simulink model "kinova"  (R2021a)
settings: Solver=FixedStepDiscrete  StartTime=0.0  StopTime=Inf  RelTol=1e-3
undefined symbols (not defined in the file): duration, gripper_finger1_joint, gripper_finger2_joint, index, joint_1, joint_2, joint_4, joint_name, model_name, my_gen3, position, velocity
libraries: robotgazebolib x28, simulink x5, rllib x1, robotlib x1
settings Model: Creator=tareksaid  LastModifiedBy=uthm

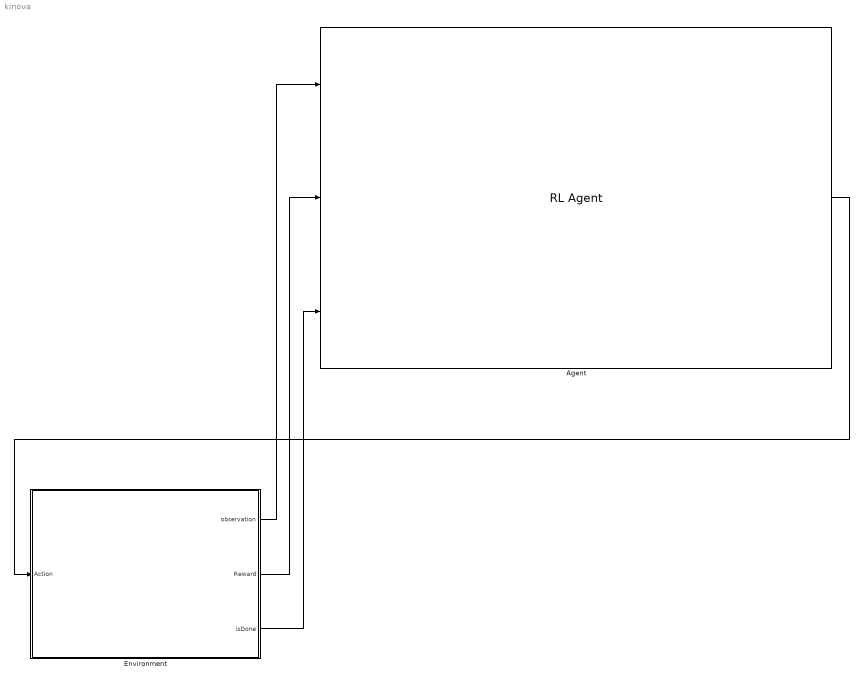
== system kinova ==
  Agent : rllib/RL Agent  Agent=Agent  ExternalActionAsInput=off  ProvideCumRwd=off  TreatAsDirectFeedthrough=on
  Environment : Subsystem
  wires:
  Environment/2(Reward) -> Agent/2
  Environment/1(observation) -> Agent/1
  Environment/3(isDone) -> Agent/3
  Agent/1 -> Environment/1(Action)

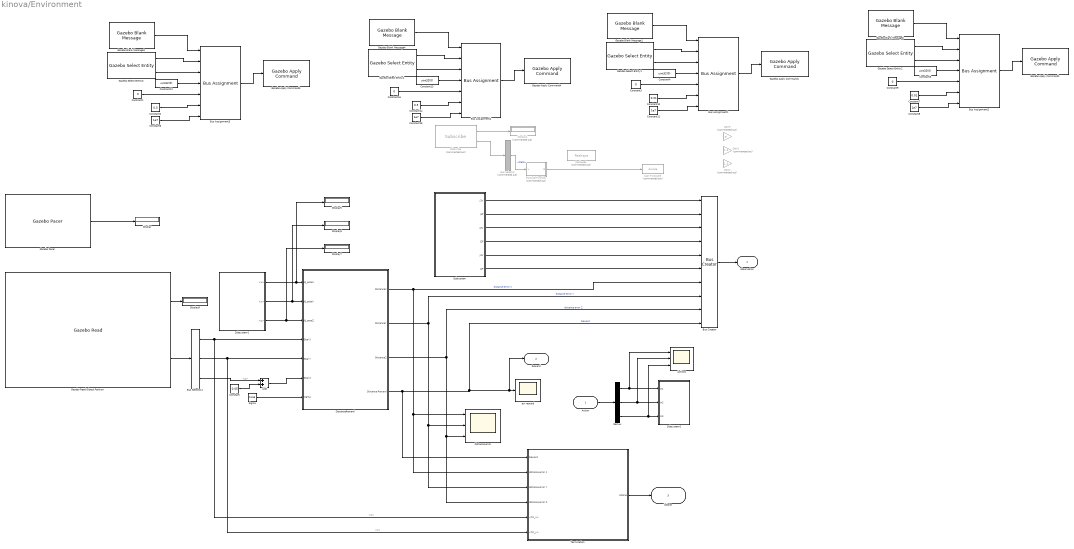
== system kinova/Environment ==
  Action : Inport
  Actions : Scope  NumInputPorts=3
  Add : Sum
  Bus Assignment1 : BusAssignment  AssignedSignals=model_name,joint_name,index,position,duration.seconds,duration.nano_seconds
  Bus Assignment2 : BusAssignment  AssignedSignals=model_name,joint_name,index,position,duration.seconds,duration.nano_seconds
  Bus Assignment3 : BusAssignment  AssignedSignals=model_name,joint_name,index,velocity,duration.seconds,duration.nano_seconds
  Bus Assignment4 : BusAssignment  AssignedSignals=model_name,joint_name,index,velocity,duration.seconds,duration.nano_seconds
  Bus Creator : BusCreator  Inputs=10
  Bus Selector : BusSelector  Commented=on  OutputSignals=Data
  Bus Selector4 : BusSelector  OutputSignals=position.x,position.y,position.z
  Cast To Double : DataTypeConversion  Commented=on  OutDataTypeStr=double
  Constant : Constant  Value=0.05
  Constant{1,3,9,16} (4 alike) : Constant  Value=0
  Constant10 : Constant  Value=0.01
  Constant{6,8,11,15} (4 alike) : Constant  Value=1e7
  Constant{4..5,12..13} (4 alike) : Constant  Value=uint32(0)
  Constant14 : Constant  Value=0.5
  Constant2 : Constant  Value=0.5
  Constant7 : Constant  Value=0.01
  Demux : Demux  Outputs=3
  Display{,5..8} (5 alike) : Display
  Display1 : Display  Commented=on
  Distance error : Scope  NumInputPorts=3
  DistanceReward : Subsystem
  Gain1 : Gain  Commented=on  Gain=1.3
  Gain2 : Gain  Commented=on  Gain=1.3
  Gain3 : Gain  Commented=on  Gain=pi
  Gazebo Apply Command1 : robotgazebolib/Gazebo Apply Command  cmdType=SetJointPosition  sampleTime=0.1
      settings: SourceProductBaseCode=RO
  Gazebo Apply Command2 : robotgazebolib/Gazebo Apply Command  cmdType=SetJointPosition  sampleTime=0.1
      settings: SourceProductBaseCode=RO
  Gazebo Apply Command3 : robotgazebolib/Gazebo Apply Command  cmdType=SetJointVelocity  sampleTime=0.1
      settings: SourceProductBaseCode=RO
  Gazebo Apply Command4 : robotgazebolib/Gazebo Apply Command  cmdType=SetJointVelocity  sampleTime=0.1
      settings: SourceProductBaseCode=RO
  Gazebo Blank Message1 : robotgazebolib/Gazebo Blank Message  msgType=SetJointPosition  sampleTime=0.1  busName='Gazebo_SL_Bus_gazebo_msgs_SetJointPosition'
      settings: SourceProductBaseCode=RO
  Gazebo Blank Message2 : robotgazebolib/Gazebo Blank Message  msgType=SetJointPosition  sampleTime=0.1  busName='Gazebo_SL_Bus_gazebo_msgs_SetJointPosition'
      settings: SourceProductBaseCode=RO
  Gazebo Blank Message3 : robotgazebolib/Gazebo Blank Message  msgType=SetJointVelocity  sampleTime=0.1  busName='Gazebo_SL_Bus_gazebo_msgs_SetJointVelocity'
      settings: SourceProductBaseCode=RO
  Gazebo Blank Message4 : robotgazebolib/Gazebo Blank Message  msgType=SetJointVelocity  sampleTime=0.1  busName='Gazebo_SL_Bus_gazebo_msgs_SetJointVelocity'
      settings: SourceProductBaseCode=RO
  Gazebo Pacer : robotgazebolib/Gazebo Pacer  ResetBehavior=Reset Gazebo simulation time and scene  SampleTime=0.1
      settings: SourceProductBaseCode=RO
  Gazebo Read Object Position : robotgazebolib/Gazebo Read  topicSource=From Gazebo  topic=/gazebo/ground_truth/world_pose/Yellow Can/link  messageType=gazebo_msgs/Pose  sampleTime=0.1
      settings: SourceProductBaseCode=RO
  Gazebo Select Entity1 : robotgazebolib/Gazebo Select Entity  modelElemName=my_gen3/gripper_finger1_joint  outputArraySize=128  OutputLabel=Joint  SelectType=Joint
      settings: SourceProductBaseCode=RO
  Gazebo Select Entity2 : robotgazebolib/Gazebo Select Entity  modelElemName=my_gen3/gripper_finger2_joint  outputArraySize=128  OutputLabel=Joint  SelectType=Joint
      settings: SourceProductBaseCode=RO
  Gazebo Select Entity3 : robotgazebolib/Gazebo Select Entity  modelElemName=my_gen3/gripper_finger1_joint  outputArraySize=128  OutputLabel=Joint  SelectType=Joint
      settings: SourceProductBaseCode=RO
  Gazebo Select Entity4 : robotgazebolib/Gazebo Select Entity  modelElemName=my_gen3/gripper_finger2_joint  outputArraySize=128  OutputLabel=Joint  SelectType=Joint
      settings: SourceProductBaseCode=RO
  MATLAB Function : MATLAB Function  Commented=on  TreatAsAtomicUnit=on
  Reshape1 : Reshape  Commented=on  OutputDimensionality=Customize  OutputDimensions=[10000,1]
  Sigma : Constant  Value=0.415
  Subscribe : robotlib/Subscribe  Commented=on  topicSource=Select from ROS network  topic=/camera/depth/image_raw  messageType=sensor_msgs/Image  SampleTime=-1  legacyBusStruct=off  messageQueueLength=1
  Subsystem : Subsystem
  Subsystem1 : Subsystem
  Subsystem2 : Subsystem
  Termination : Subsystem
  avr reward : Scope
  observation : Outport
  Reward : Outport  Port=2
  isDone : Outport  Port=3  VectorParamsAs1DForOutWhenUnconnected=off
  wires:
  Bus Creator/1 -> observation/1
  Termination/1(isDone) -> isDone/1
  Gazebo Pacer/1 -> Display/1
  DistanceReward/1(DistanceX) -> Bus Creator/7, Termination/2(distance error X), Distance error/1  "distance error X"
  Bus Selector4/2 -> Termination/6(<tin_y>), DistanceReward/5(Goal Y)  "<y>"
  DistanceReward/4(Distance Reward) -> Termination/1(Reward), Bus Creator/10, avr reward/1, Reward/1  "Reward"
  DistanceReward/2(DistanceY) -> Bus Creator/8, Termination/3(distance error Y), Distance error/2  "distance error Y"
  DistanceReward/3(DistanceZ) -> Bus Creator/9, Termination/4(distance error Z), Distance error/3  "distance error Z"
  Sigma/1 -> DistanceReward/7(sigma)
  Action/1 -> Demux/1
  Demux/2 -> Actions/2, Subsystem2/2(In2)
  Demux/3 -> Actions/3, Subsystem2/3(In3)
  Demux/1 -> Actions/1, Subsystem2/1(In1)
  Gazebo Read Object Position/1 -> Display8/1
  Gazebo Read Object Position/2 -> Bus Selector4/1
  Bus Selector4/1 -> Termination/5(<tin_x>), DistanceReward/4(Goal X)  "<x>"
  Subsystem/1(J1V) -> Bus Creator/1
  Subsystem/2(J1P) -> Bus Creator/2
  Subsystem/3(J2V) -> Bus Creator/3
  Subsystem/4(J2P) -> Bus Creator/4
  Subsystem/5(J4V) -> Bus Creator/5
  Subsystem/6(J4P) -> Bus Creator/6
  Subsystem1/2(<y>) -> Display6/1, DistanceReward/2(j8_poseY)
  Subsystem1/3(<z>) -> Display7/1, DistanceReward/3(j8_poseZ)
  Subsystem1/1(<x>) -> Display5/1, DistanceReward/1(j8_poseX)
  Subscribe/2 -> Bus Selector/1
  Bus Selector/1 -> MATLAB Function/1(u)  "<Data>"
  Subscribe/1 -> Display1/1
  MATLAB Function/1(D) -> Cast To Double/1
  Bus Selector4/3 -> Add/1  "<z>"
  Constant/1 -> Add/2
  Add/1 -> DistanceReward/6(Goal Z)
  Bus Assignment3/1 -> Gazebo Apply Command3/1
  Gazebo Select Entity3/2 -> Bus Assignment3/3
  Gazebo Select Entity3/1 -> Bus Assignment3/2
  Constant12/1 -> Bus Assignment3/4
  Constant16/1 -> Bus Assignment4/5
  Constant6/1 -> Bus Assignment3/7
  Constant2/1 -> Bus Assignment3/6
  Gazebo Blank Message3/1 -> Bus Assignment3/1
  Constant1/1 -> Bus Assignment3/5
  Bus Assignment4/1 -> Gazebo Apply Command4/1
  Constant15/1 -> Bus Assignment4/7
  Gazebo Blank Message4/1 -> Bus Assignment4/1
  Gazebo Select Entity4/1 -> Bus Assignment4/2
  Gazebo Select Entity4/2 -> Bus Assignment4/3
  Constant13/1 -> Bus Assignment4/4
  Constant14/1 -> Bus Assignment4/6
  Constant7/1 -> Bus Assignment2/6
  Constant5/1 -> Bus Assignment2/4
  Gazebo Select Entity2/2 -> Bus Assignment2/3
  Gazebo Select Entity2/1 -> Bus Assignment2/2
  Gazebo Blank Message2/1 -> Bus Assignment2/1
  Constant8/1 -> Bus Assignment2/7
  Bus Assignment2/1 -> Gazebo Apply Command2/1
  Constant3/1 -> Bus Assignment1/5
  Gazebo Blank Message1/1 -> Bus Assignment1/1
  Constant10/1 -> Bus Assignment1/6
  Constant11/1 -> Bus Assignment1/7
  Constant9/1 -> Bus Assignment2/5
  Constant4/1 -> Bus Assignment1/4
  Gazebo Select Entity1/1 -> Bus Assignment1/2
  Gazebo Select Entity1/2 -> Bus Assignment1/3
  Bus Assignment1/1 -> Gazebo Apply Command1/1

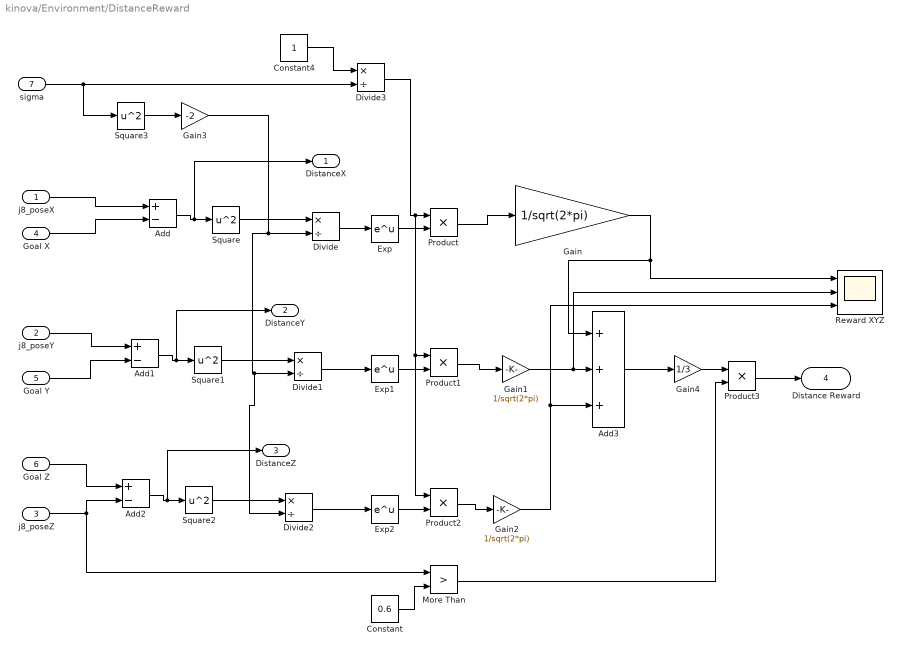
== system kinova/Environment/DistanceReward ==
  j8_poseX : Inport
  j8_poseY : Inport  Port=2
  j8_poseZ : Inport  Port=3
  Goal X : Inport  Port=4
  Goal Y : Inport  Port=5
  Goal Z : Inport  Port=6
  sigma : Inport  Port=7
  Add : Sum  Inputs=+-
  Add1 : Sum  Inputs=+-
  Add2 : Sum  Inputs=+-
  Add3 : Sum  Inputs=+++
  Constant : Constant  Value=0.6
  Constant4 : Constant
  Divide{,1..3} (4 alike) : Product  Inputs=*/
  Exp : Math  SaturateOnIntegerOverflow=on
  Exp1 : Math  SaturateOnIntegerOverflow=on
  Exp2 : Math  SaturateOnIntegerOverflow=on
  Gain : Gain  Gain=1/sqrt(2*pi)
  Gain1 : Gain  Gain=1/sqrt(2*pi)
  Gain2 : Gain  Gain=1/sqrt(2*pi)
  Gain3 : Gain  Gain=-2
  Gain4 : Gain  Gain=1/3
  More Than : RelationalOperator  Operator=>  OutDataTypeStr=boolean  RndMeth=Simplest
  Product{,1..3} (4 alike) : Product
  Reward XYZ : Scope  NumInputPorts=3
  Square{,1..3} (4 alike) : Math  Operator=square  SaturateOnIntegerOverflow=on
  DistanceX : Outport
  DistanceY : Outport  Port=2
  DistanceZ : Outport  Port=3
  Distance Reward : Outport  Port=4
  wires:
  Goal X/1 -> Add/2
  j8_poseX/1 -> Add/1
  Divide/1 -> Exp/1
  Square/1 -> Divide/1
  Add/1 -> DistanceX/1, Square/1
  Add1/1 -> Square1/1, DistanceY/1
  Square1/1 -> Divide1/1
  Divide1/1 -> Exp1/1
  j8_poseY/1 -> Add1/1
  Goal Y/1 -> Add1/2
  Divide2/1 -> Exp2/1
  Square2/1 -> Divide2/1
  Add2/1 -> DistanceZ/1, Square2/1
  Goal Z/1 -> Add2/1
  Gain1/1 -> Reward XYZ/2, Add3/2
  Gain/1 -> Add3/1, Reward XYZ/1
  Gain2/1 -> Add3/3, Reward XYZ/3
  Square3/1 -> Gain3/1
  Constant4/1 -> Divide3/1
  sigma/1 -> Divide3/2, Square3/1
  Exp/1 -> Product/2
  Exp1/1 -> Product1/2
  Exp2/1 -> Product2/2
  Divide3/1 -> Product2/1, Product1/1, Product/1
  Product/1 -> Gain/1
  Product1/1 -> Gain1/1
  Product2/1 -> Gain2/1
  Gain3/1 -> Divide/2, Divide2/2, Divide1/2
  Add3/1 -> Gain4/1
  More Than/1 -> Product3/2
  Constant/1 -> More Than/2
  j8_poseZ/1 -> More Than/1, Add2/2
  Gain4/1 -> Product3/1
  Product3/1 -> Distance Reward/1

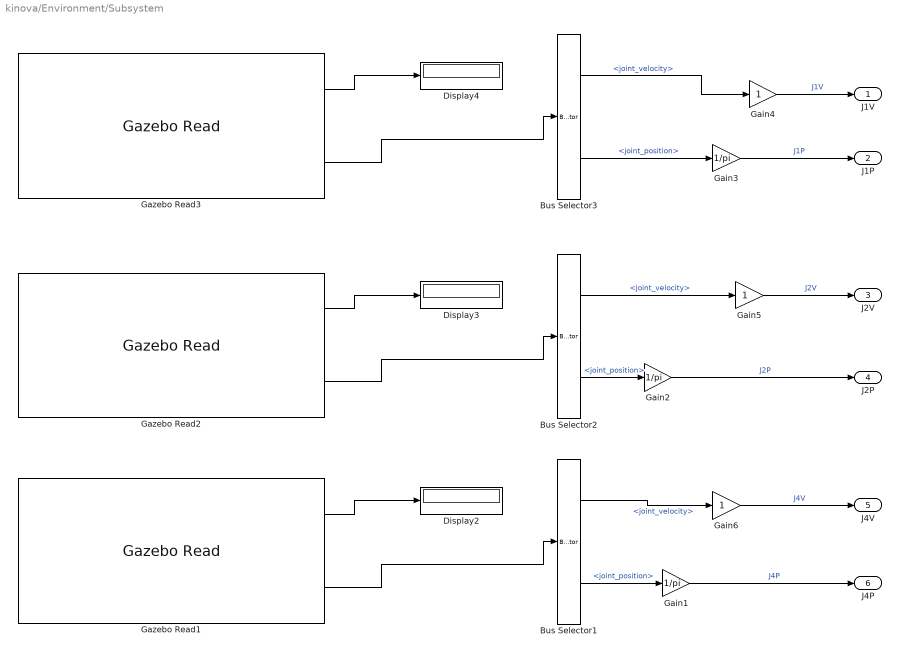
== system kinova/Environment/Subsystem ==
  Bus Selector1 : BusSelector  OutputSignals=joint_velocity,joint_position
  Bus Selector2 : BusSelector  OutputSignals=joint_velocity,joint_position
  Bus Selector3 : BusSelector  OutputSignals=joint_velocity,joint_position
  Display2 : Display
  Display3 : Display
  Display4 : Display
  Gain1 : Gain  Gain=1/pi
  Gain2 : Gain  Gain=1/pi
  Gain3 : Gain  Gain=1/pi
  Gain4 : Gain
  Gain5 : Gain
  Gain6 : Gain
  Gazebo Read1 : robotgazebolib/Gazebo Read  topicSource=From Gazebo  topic=/gazebo/ground_truth/joint_state/my_gen3/joint_4  messageType=gazebo_msgs/JointState  sampleTime=0.1
      settings: SourceProductBaseCode=RO
  Gazebo Read2 : robotgazebolib/Gazebo Read  topicSource=From Gazebo  topic=/gazebo/ground_truth/joint_state/my_gen3/joint_2  messageType=gazebo_msgs/JointState  sampleTime=0.1
      settings: SourceProductBaseCode=RO
  Gazebo Read3 : robotgazebolib/Gazebo Read  topicSource=From Gazebo  topic=/gazebo/ground_truth/joint_state/my_gen3/joint_1  messageType=gazebo_msgs/JointState  sampleTime=0.1
      settings: SourceProductBaseCode=RO
  J1V : Outport
  J1P : Outport  Port=2
  J2V : Outport  Port=3
  J2P : Outport  Port=4
  J4V : Outport  Port=5
  J4P : Outport  Port=6
  wires:
  Bus Selector2/1 -> Gain5/1  "<joint_velocity>"
  Gain3/1 -> J1P/1  "J1P"
  Gazebo Read2/1 -> Display3/1
  Bus Selector1/1 -> Gain6/1  "<joint_velocity>"
  Gazebo Read1/1 -> Display2/1
  Bus Selector2/2 -> Gain2/1  "<joint_position>"
  Gazebo Read3/1 -> Display4/1
  Bus Selector1/2 -> Gain1/1  "<joint_position>"
  Gazebo Read1/2 -> Bus Selector1/1
  Gazebo Read2/2 -> Bus Selector2/1
  Bus Selector3/2 -> Gain3/1  "<joint_position>"
  Gazebo Read3/2 -> Bus Selector3/1
  Bus Selector3/1 -> Gain4/1  "<joint_velocity>"
  Gain5/1 -> J2V/1  "J2V"
  Gain6/1 -> J4V/1  "J4V"
  Gain4/1 -> J1V/1  "J1V"
  Gain2/1 -> J2P/1  "J2P"
  Gain1/1 -> J4P/1  "J4P"

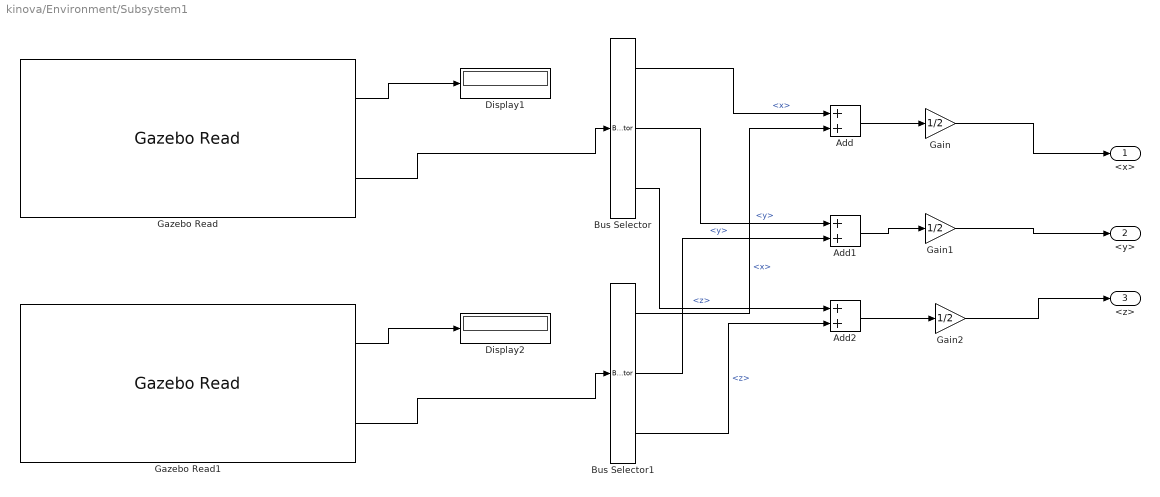
== system kinova/Environment/Subsystem1 ==
  Add : Sum
  Add1 : Sum
  Add2 : Sum
  Bus Selector : BusSelector  OutputSignals=world_pose.position.x,world_pose.position.y,world_pose.position.z
  Bus Selector1 : BusSelector  OutputSignals=world_pose.position.x,world_pose.position.y,world_pose.position.z
  Display1 : Display
  Display2 : Display
  Gain : Gain  Gain=1/2
  Gain1 : Gain  Gain=1/2
  Gain2 : Gain  Gain=1/2
  Gazebo Read : robotgazebolib/Gazebo Read  topicSource=From Gazebo  topic=/gazebo/ground_truth/joint_state/my_gen3/gripper_finger1_joint  messageType=gazebo_msgs/JointState  sampleTime=0.1
      settings: SourceProductBaseCode=RO
  Gazebo Read1 : robotgazebolib/Gazebo Read  topicSource=From Gazebo  topic=/gazebo/ground_truth/joint_state/my_gen3/gripper_finger2_joint  messageType=gazebo_msgs/JointState  sampleTime=0.1
      settings: SourceProductBaseCode=RO
  <x> : Outport
  <y> : Outport  Port=2
  <z> : Outport  Port=3
  wires:
  Gazebo Read/2 -> Bus Selector/1
  Gazebo Read/1 -> Display1/1
  Gazebo Read1/1 -> Display2/1
  Gazebo Read1/2 -> Bus Selector1/1
  Bus Selector/1 -> Add/1  "<x>"
  Bus Selector1/1 -> Add/2  "<x>"
  Bus Selector/2 -> Add1/1  "<y>"
  Bus Selector1/2 -> Add1/2  "<y>"
  Bus Selector/3 -> Add2/1  "<z>"
  Bus Selector1/3 -> Add2/2  "<z>"
  Add/1 -> Gain/1
  Add1/1 -> Gain1/1
  Add2/1 -> Gain2/1
  Gain/1 -> <x>/1
  Gain1/1 -> <y>/1
  Gain2/1 -> <z>/1

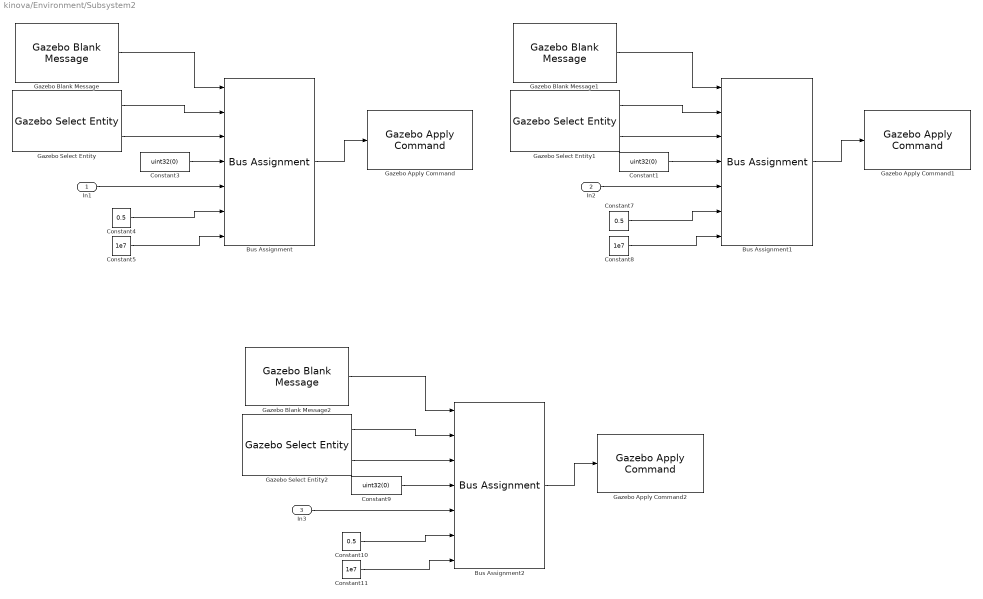
== system kinova/Environment/Subsystem2 ==
  In1 : Inport
  In2 : Inport  Port=2
  In3 : Inport  Port=3
  Bus Assignment : BusAssignment  AssignedSignals=model_name,joint_name,index,velocity,duration.seconds,duration.nano_seconds
  Bus Assignment1 : BusAssignment  AssignedSignals=model_name,joint_name,index,velocity,duration.seconds,duration.nano_seconds
  Bus Assignment2 : BusAssignment  AssignedSignals=model_name,joint_name,index,velocity,duration.seconds,duration.nano_seconds
  Constant1 : Constant  Value=uint32(0)
  Constant10 : Constant  Value=0.5
  Constant11 : Constant  Value=1e7
  Constant3 : Constant  Value=uint32(0)
  Constant4 : Constant  Value=0.5
  Constant5 : Constant  Value=1e7
  Constant7 : Constant  Value=0.5
  Constant8 : Constant  Value=1e7
  Constant9 : Constant  Value=uint32(0)
  Gazebo Apply Command : robotgazebolib/Gazebo Apply Command  cmdType=SetJointVelocity  sampleTime=0.1
      settings: SourceProductBaseCode=RO
  Gazebo Apply Command1 : robotgazebolib/Gazebo Apply Command  cmdType=SetJointVelocity  sampleTime=0.1
      settings: SourceProductBaseCode=RO
  Gazebo Apply Command2 : robotgazebolib/Gazebo Apply Command  cmdType=SetJointVelocity  sampleTime=0.1
      settings: SourceProductBaseCode=RO
  Gazebo Blank Message : robotgazebolib/Gazebo Blank Message  msgType=SetJointVelocity  sampleTime=0.1  busName='Gazebo_SL_Bus_gazebo_msgs_SetJointVelocity'
      settings: SourceProductBaseCode=RO
  Gazebo Blank Message1 : robotgazebolib/Gazebo Blank Message  msgType=SetJointVelocity  sampleTime=0.1  busName='Gazebo_SL_Bus_gazebo_msgs_SetJointVelocity'
      settings: SourceProductBaseCode=RO
  Gazebo Blank Message2 : robotgazebolib/Gazebo Blank Message  msgType=SetJointVelocity  sampleTime=0.1  busName='Gazebo_SL_Bus_gazebo_msgs_SetJointVelocity'
      settings: SourceProductBaseCode=RO
  Gazebo Select Entity : robotgazebolib/Gazebo Select Entity  modelElemName=my_gen3/joint_1  outputArraySize=128  OutputLabel=Joint  SelectType=Joint
      settings: SourceProductBaseCode=RO
  Gazebo Select Entity1 : robotgazebolib/Gazebo Select Entity  modelElemName=my_gen3/joint_2  outputArraySize=128  OutputLabel=Joint  SelectType=Joint
      settings: SourceProductBaseCode=RO
  Gazebo Select Entity2 : robotgazebolib/Gazebo Select Entity  modelElemName=my_gen3/joint_4  outputArraySize=128  OutputLabel=Joint  SelectType=Joint
      settings: SourceProductBaseCode=RO
  wires:
  Gazebo Blank Message/1 -> Bus Assignment/1
  Constant7/1 -> Bus Assignment1/6
  Bus Assignment1/1 -> Gazebo Apply Command1/1
  Gazebo Select Entity1/2 -> Bus Assignment1/3
  Gazebo Select Entity/2 -> Bus Assignment/3
  Bus Assignment2/1 -> Gazebo Apply Command2/1
  Constant4/1 -> Bus Assignment/6
  Constant10/1 -> Bus Assignment2/6
  Bus Assignment/1 -> Gazebo Apply Command/1
  Gazebo Blank Message1/1 -> Bus Assignment1/1
  In1/1 -> Bus Assignment/5
  Gazebo Blank Message2/1 -> Bus Assignment2/1
  Constant11/1 -> Bus Assignment2/7
  Constant1/1 -> Bus Assignment1/4
  In2/1 -> Bus Assignment1/5
  Gazebo Select Entity/1 -> Bus Assignment/2
  Gazebo Select Entity2/1 -> Bus Assignment2/2
  Constant9/1 -> Bus Assignment2/4
  Gazebo Select Entity1/1 -> Bus Assignment1/2
  Constant5/1 -> Bus Assignment/7
  Constant8/1 -> Bus Assignment1/7
  Gazebo Select Entity2/2 -> Bus Assignment2/3
  Constant3/1 -> Bus Assignment/4
  In3/1 -> Bus Assignment2/5

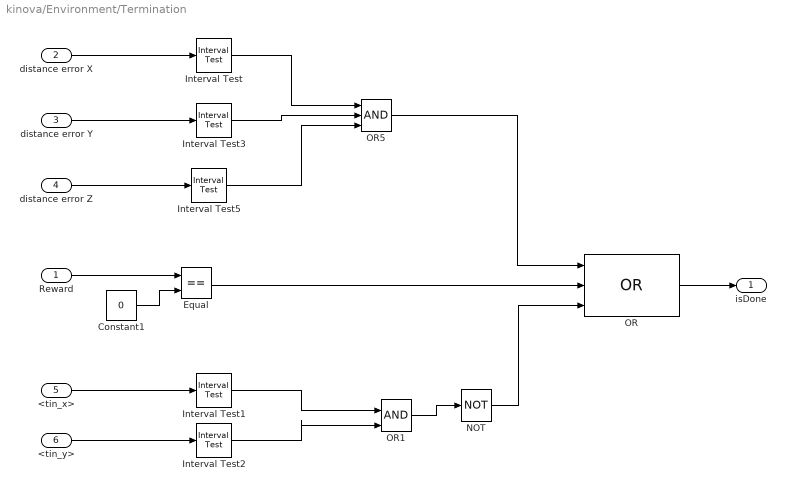
== system kinova/Environment/Termination ==
  Reward : Inport
  distance error X : Inport  Port=2
  distance error Y : Inport  Port=3
  distance error Z : Inport  Port=4
  <tin_x> : Inport  Port=5
  <tin_y> : Inport  Port=6
  Constant1 : Constant  Value=0
  Equal : RelationalOperator  Operator===  OutDataTypeStr=boolean  RndMeth=Simplest
  Interval Test : simulink/Logic and Bit Operations/Interval Test  IntervalClosedRight=on  uplimit=0.01  IntervalClosedLeft=on  lowlimit=-0.01  OutDataTypeStr=boolean
  Interval Test1 : simulink/Logic and Bit Operations/Interval Test  IntervalClosedRight=on  uplimit=0.7  IntervalClosedLeft=on  lowlimit=0.05  OutDataTypeStr=boolean
  Interval Test2 : simulink/Logic and Bit Operations/Interval Test  IntervalClosedRight=on  uplimit=0.5  IntervalClosedLeft=on  lowlimit=-0.5  OutDataTypeStr=boolean
  Interval Test3 : simulink/Logic and Bit Operations/Interval Test  IntervalClosedRight=on  uplimit=0.01  IntervalClosedLeft=on  lowlimit=-0.01  OutDataTypeStr=boolean
  Interval Test5 : simulink/Logic and Bit Operations/Interval Test  IntervalClosedRight=on  uplimit=0.01  IntervalClosedLeft=on  lowlimit=-0.01  OutDataTypeStr=boolean
  NOT : Logic  Operator=NOT  IconShape=distinctive  AllPortsSameDT=off  OutDataTypeStr=boolean
  OR : Logic  Operator=OR  Inputs=3  IconShape=distinctive  AllPortsSameDT=off  OutDataTypeStr=boolean
  OR1 : Logic  IconShape=distinctive  AllPortsSameDT=off  OutDataTypeStr=boolean
  OR5 : Logic  Inputs=3  IconShape=distinctive  AllPortsSameDT=off  OutDataTypeStr=boolean
  isDone : Outport  VectorParamsAs1DForOutWhenUnconnected=off
  wires:
  Interval Test/1 -> OR5/1
  Interval Test3/1 -> OR5/2
  Interval Test5/1 -> OR5/3
  OR5/1 -> OR/1
  OR/1 -> isDone/1
  Reward/1 -> Equal/1
  Constant1/1 -> Equal/2
  distance error Z/1 -> Interval Test5/1
  distance error Y/1 -> Interval Test3/1
  distance error X/1 -> Interval Test/1
  Interval Test1/1 -> OR1/1
  Interval Test2/1 -> OR1/2
  Equal/1 -> OR/2
  OR1/1 -> NOT/1
  <tin_x>/1 -> Interval Test1/1
  <tin_y>/1 -> Interval Test2/1
  NOT/1 -> OR/3

== matlab function kinova/Environment/MATLAB Function ==
  data: u input; D output
function D = fcn(u)

D = u(3:4:end);
% D = reshape(Ds, 10000, 1)';
